simulink model "speedDistanceRegulator__impl"  (R2017b)
settings: Solver=FixedStepDiscrete  StartTime=0.0  StopTime=10.0  FixedStep=1.0  RelTol=1e-3
model mask{kp=kp, kd=kd, ki=ki}
PreLoadFcn:
  | sl_refresh_customizations
  | enum_Simulink
  | simulinkExportUnitCs
  | ACC_Parameters
  | ACCData
InitFcn:
  | checkUnitMismatch
model workspace (MAT data in the model file):
  ESD_URL = 'http://127.0.0.1:63320/node?ref=r%3Af6839c77-5b9d-441b-9a46-8668f7352d69%28A_ACC._50_ImplementationDefinitionHeterogeneous%29%2F1192123807590925362'
  ModelMaskData(1).paramName = 'kp'
  ModelMaskData(1).paramType = 'double'
  ModelMaskData(1).promptString = 'kp(datatype: double, unit:)'
  ModelMaskData(2).paramName = 'kd'
  ModelMaskData(2).paramType = 'double'
  ModelMaskData(2).promptString = 'kd(datatype: double, unit:)'
  ModelMaskData(3).paramName = 'ki'
  ModelMaskData(3).paramType = 'double'
  ModelMaskData(3).promptString = 'ki(datatype: double, unit:)'
  kd = Simulink.Parameter
  kd.Value = 0
  kd.DataType = 'double'
  kd.Dimensions = [1 1]
  ki = Simulink.Parameter
  ki.Value = 0
  ki.DataType = 'double'
  ki.Dimensions = [1 1]
  kp = Simulink.Parameter
  kp.Value = 0
  kp.DataType = 'double'
  kp.Dimensions = [1 1]
settings Model: ParameterArgumentNames=kp,kd,ki  Creator=eh6qym  LastModifiedBy=eh6qym
settings OptimizationCC: DefaultParameterBehavior=Inlined  PassReuseOutputArgsAs=Individual arguments  ZeroExternalMemoryAtStartup=off
settings DebuggingCC: SignalRangeChecking=error  InheritedTsInSrcMsg=none  ParameterTunabilityLossMsg=error
settings SFSimCC: MATLABDynamicMemAlloc=off
settings RTWCC: SystemTargetFile=esd_ert.tlc  GenCodeOnly=on  TemplateMakefile=ert_default_tmf  Description=CSD  GenerateReport=on  IncludeHyperlinkInReport=on  LaunchReport=on  GenerateTraceInfo=on  GenerateTraceReport=on  GenerateTraceReportSl=on  GenerateTraceReportSf=on  GenerateTraceReportEml=on
settings CodeAppCC: ForceParamTrailComments=on  IgnoreCustomStorageClasses=off  OperatorAnnotations=on  SimulinkDataObjDesc=on  SFDataObjDesc=on  InsertBlockDesc=on
settings STFCustomTargetCC: TargetLangStandard=C99 (ISO)  MultiwordLength=256  GenerateSampleERTMain=on  IncludeMdlTerminateFcn=off  CombineOutputUpdateFcns=on  CombineSignalStateStructs=on  SuppressErrorStatus=on  ERTCustomFileBanners=on  MultiInstanceERTCode=on  CodeInterfacePackaging=Reusable function  SupportContinuousTime=off  SupportNonInlinedSFcns=off  RemoveDisableFunc=on  RemoveResetFunc=on  MATLABClassNameForMDSCustomization=Simulink.SoftwareTarget.ERTCustomization  GRTInterface=off  SystemTargetFile=esd_ert.tlc
settings ERTTargetCC: TargetLangStandard=C99 (ISO)  GenerateSampleERTMain=on  ParMdlRefBuildCompliant=off  CompOptLevelCompliant=off  ConcurrentExecutionCompliant=off  IncludeMdlTerminateFcn=off  CombineSignalStateStructs=on  SuppressErrorStatus=on  MultiInstanceERTCode=on  CodeInterfacePackaging=Reusable function  RemoveDisableFunc=on  ModelStepFunctionPrototypeControlCompliant=off  CPPClassGenCompliant=off  UseToolchainInfoCompliant=off  InlinedParameterPlacement=NonHierarchical  ERTCustomFileTemplate=example_file_process.tlc

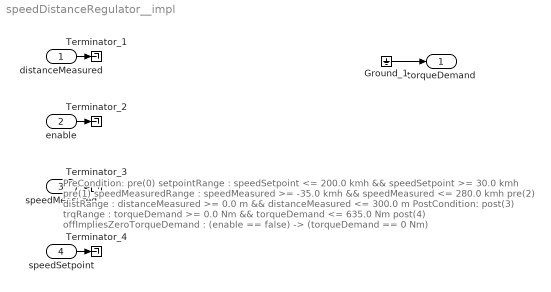
== system speedDistanceRegulator__impl ==
  note: PreCondition:
      | pre(0) setpointRange :   speedSetpoint <= 200.0 kmh && speedSetpoint >= 30.0 kmh
      | pre(1) speedMeasuredRange :   speedMeasured >= -35.0 kmh && speedMeasured <= 280.0 kmh
      | pre(2) distRange :   distanceMeasured >= 0.0 m && distanceMeasured <= 300.0 m
      | PostCondition:
      | post(3) trqRange :   torqueDemand >= 0.0 Nm && torqueDemand <= 635.0 Nm
      | post(4) offImpliesZeroTorqueDemand :   (enable == false) -> (torqueDemand == 0 Nm)
  distanceMeasured : Inport  OutDataTypeStr=double  Unit=m
      settings: AttributesFormatString=(m)
  enable : Inport  Port=2  OutDataTypeStr=boolean
  speedMeasured : Inport  Port=3  OutDataTypeStr=double  Unit=kmh
      settings: AttributesFormatString=(kmh)
  speedSetpoint : Inport  Port=4  OutDataTypeStr=double  Unit=kmh
      settings: AttributesFormatString=(kmh)
  Ground_1 : Ground
  Terminator_{1..4} (4 alike) : Terminator
  torqueDemand : Outport  OutDataTypeStr=double  Unit=Nm
      settings: AttributesFormatString=(Nm)
  wires:
  distanceMeasured/1 -> Terminator_1/1
  enable/1 -> Terminator_2/1
  speedMeasured/1 -> Terminator_3/1
  speedSetpoint/1 -> Terminator_4/1
  Ground_1/1 -> torqueDemand/1
